simulink model "mbed_nucleo_f303_counter"  (R2015a)
settings: Solver=FixedStepDiscrete  SolverMode=SingleTasking  StartTime=0.0  StopTime=10.0  FixedStep=1  RelTol=1e-3
libraries: mbed_targets_stm_nucleo_f303 x2, mbed_lib x2, simulink x1, mbed_targets_stm_disco_f407 x1
settings Model: Creator=Stuv  LastModifiedBy=Stuv
settings OptimizationCC: OptimizeModelRefInitCode=on  LifeSpan=1
settings HardwareCC: ProdLargestAtomicInteger=Long  ProdLargestAtomicFloat=Double  ProdEndianess=LittleEndian  ProdHWDeviceType=ARM Compatible->ARM Cortex
settings RTWCC: SystemTargetFile=mbed.tlc  TemplateMakefile=mbed.tmf  Description=Mbed Target (Embedded Target)  TargetLang=C++
settings CodeAppCC: IgnoreCustomStorageClasses=off
settings STFCustomTargetCC: CombineOutputUpdateFcns=on  SupportContinuousTime=off  SupportVariableSizeSignals=off  SystemTargetFile=mbed.tlc
settings ERTTargetCC: SupportContinuousTime=off  SupportVariableSizeSignals=off  ERTCustomFileTemplate=mbed_file_process.tlc

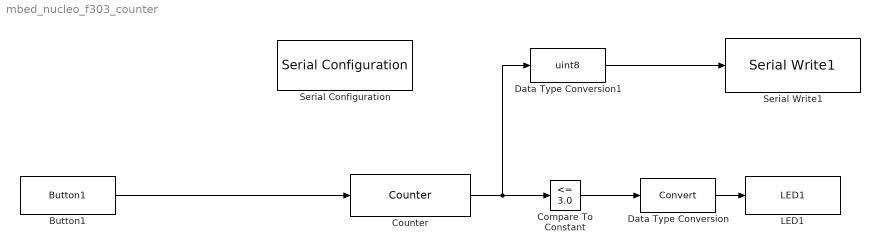
== system mbed_nucleo_f303_counter ==
  Button1 : mbed_targets_stm_nucleo_f303/Button1  Parameter1=0
  Compare To Constant : simulink/Logic and Bit Operations/Compare To Constant  relop=<=  const=3.0  OutDataTypeStr=boolean
  Counter : mbed_targets_stm_disco_f407/Counter  TimerNumber=4  InputChannel=TI1 falling  TiPort=A  TiPin=11  TiPupd=PullUp  MaxCnt=6  Interrupt=no interrupt generation  RstEnable=on
  Data Type Conversion : DataTypeConversion
  Data Type Conversion1 : DataTypeConversion  OutDataTypeStr=uint8
  LED1 : mbed_targets_stm_nucleo_f303/LED1  Parameter1=0
  Serial Configuration : mbed_lib/Serial/Serial Configuration  SerialPort=1  TXPort=A  TXPin=2  RXPort=A  RXPin=3  BaudRate=115200
  Serial Write1 : mbed_lib/Serial/Serial Write1  SerialPort=1  numData=off  SampleTime=-1
  wires:
  Button1/1 -> Counter/1
  Counter/1 -> Data Type Conversion1/1, Compare To Constant/1
  Compare To Constant/1 -> Data Type Conversion/1
  Data Type Conversion/1 -> LED1/1
  Data Type Conversion1/1 -> Serial Write1/1
